simulink model "test_enum_model"  (R2023b)
settings: Solver=VariableStepAuto  StartTime=0.0  StopTime=10.0  RelTol=1e-3
values from neighbouring files (symbols this model uses):
  Signal_Enum : value not decoded    [my_data.sldd]
libraries: simulink x2
settings Model: DataDictionary=my_data.sldd  Creator=fy153  LastModifiedBy=fy153

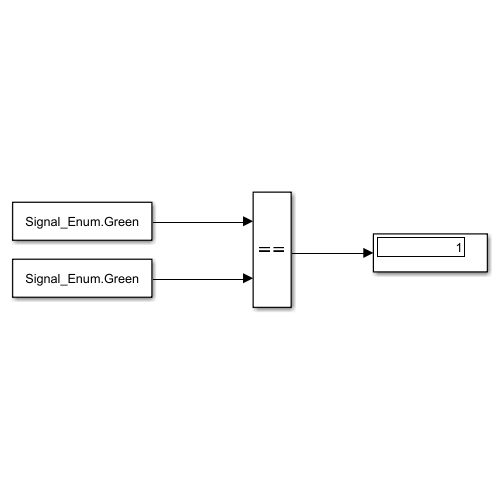
[thumbnail: Simulink's stored preview of the top-level diagram]
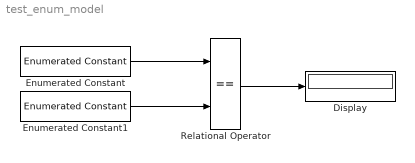
== system test_enum_model ==
  Display : Display
  Enumerated Constant : simulink/Sources/Enumerated Constant  OutDataTypeStr=Enum: Signal_Enum  Value=Signal_Enum.Green  SampleTime=inf
  Enumerated Constant1 : simulink/Sources/Enumerated Constant  OutDataTypeStr=Enum: Signal_Enum  Value=Signal_Enum.Green  SampleTime=inf
  Relational Operator : RelationalOperator  Operator===  OutDataTypeStr=boolean  RndMeth=Simplest  InputSameDT=off
  wires:
  Enumerated Constant/1 -> Relational Operator/1
  Enumerated Constant1/1 -> Relational Operator/2
  Relational Operator/1 -> Display/1
